simulink model "Runnig_sum"  (R2018a)
settings: Solver=VariableStepAuto  StartTime=0.0  StopTime=1  RelTol=1e-3
settings Model: Creator=HP  LastModifiedBy=HP

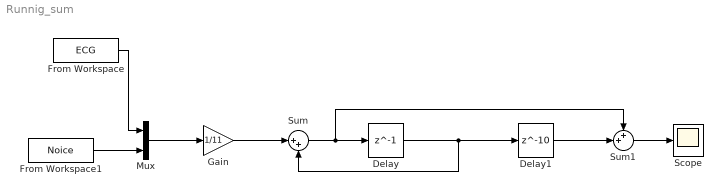
== system Runnig_sum ==
  Delay : Delay  DelayLength=1  InitialCondition=0
  Delay1 : Delay  DelayLength=10  InitialCondition=0
  From Workspace : FromWorkspace  VariableName=ECG  SampleTime=0
  From Workspace1 : FromWorkspace  VariableName=Noice  SampleTime=0
  Gain : Gain  Gain=1/11
  Mux : Mux  Inputs=2
  Scope : Scope
  Sum : Sum  Inputs=|++
  Sum1 : Sum  Inputs=++|
  wires:
  Delay/1 -> Sum/2, Delay1/1
  Delay1/1 -> Sum1/2
  Sum/1 -> Sum1/1, Delay/1
  Gain/1 -> Sum/1
  From Workspace1/1 -> Mux/2
  From Workspace/1 -> Mux/1
  Mux/1 -> Gain/1
  Sum1/1 -> Scope/1
